simulink model "HEVminiproject"  (R2026a)
settings: configuration reference "VehicleVariable" (kept outside this file)
StartFcn:
  | %tic
StopFcn:
  | %toc
model workspace (MAT data in the model file):
  ExtDrvCmdsSwitch : Simulink.Parameter (value not decoded)
  ExtDrvRefSwitch : Simulink.Parameter (value not decoded)
  ExtEnvSwitch : Simulink.Parameter (value not decoded)
  ExtGndSwitch : Simulink.Parameter (value not decoded)
symbols that are objects in the model workspace (value not decoded): ExtDrvCmdsSwitch, ExtDrvRefSwitch, ExtEnvSwitch, ExtGndSwitch
undefined symbols (not defined in the file): AmbTemp, BaroPress, CtrlTcuInitGear, CurvGradRef, CurvRef, DCM, DriverAeroRes, DriverDrivelineRes, DriverInitialGear, DriverPreviewDist, DriverRollRes, DriverShiftTime, DriverTimeConst, DriverTractiveForce, EnvAbsPrs, EnvAirTemp, EnvGrvty, EnvNomFrictionScaling, EnvNominalGrade, EnvScnFrictionMap, EnvScnFrictionMapXBpts, EnvScnFrictionMapYBpts, EnvScnHeightMap, EnvScnHeightMapXBpts, EnvScnHeightMapYBpts, EnvWindVelX, EnvWindVelY, EnvWindVelZ, Gnd, Grade, HazzardCmd, HighBeamCmd, lambda_mux, LeftSignalCmd, LngRef, LowBeamCmd, LtrRef, PhiRef, PlntThrCabRelHInit, PlntThrRefrigPinit, PlntVehDstCGRearAxl, PlntVehInitYawAng, PlntVehMass, PlntVehTrckWdth, PlntVehYawMomentInertia, PlntWhlLdRadiusFrnt, PlntWhlLdRadiusRear, PsiRef, RightSignalCmd, Sim3dSensor, Wind, XRef, YRef, Z
libraries: simulink x28, autolibutils x5, autolibsharedcommon x5, vehdynlibviscommon x4, vehdynlibdriver x2, sim3dgroundtruthsensorlib x2, autolibshared x2, sl3dlib x1, sharedtransform x1, sim3dlib x1
(part 4 of 5)

== system HEVminiproject/Environment/Varying Friction/Varying Friction ==
  InertFrm : Inport
  Cg : Inport  Port=2
  Bus Creator2 : BusCreator  Inputs=4
  Bus Selector : BusSelector  OutputSignals=FrntAxl.Lft.Disp.X,FrntAxl.Rght.Disp.X,RearAxl.Lft.Disp.X,RearAxl.Rght.Disp.X
  Bus Selector1 : BusSelector  OutputSignals=FrntAxl.Lft.Disp.Y,FrntAxl.Rght.Disp.Y,RearAxl.Lft.Disp.Y,RearAxl.Rght.Disp.Y
  Demux1 : Demux
  Road Track Friction : Subsystem  mask(Road Track Friction){surface_popup=Split friction coefficient scaling factor, lambda_g=EnvNomFrictionScaling, lambda_r=.6, r_x0=175, r_y0=-100, r_xw=1000, r_yw=500, aMode=2}
      mask prompts: surface_popup "Type of surface:"; lambda_g "Scaling factor for the friction coefficient of ground, lambda_g :"; lambda_r "Scaling factor for the friction coefficient of rectangular surface, lambda_r :"; r_x0 "X coordinate of lower left corner of rectangular surface, r_x0 [m]:"; r_y0 "Y coordinate of lower left corner of rectangular surface, r_y0 [m]:"; r_xw "Rectangular surface width in X direction, r_xw [m]:"; r_yw "Rectangular surface width in Y direction, r_yw [m]:"
      mask init:
      | % Scaling factor for the friction coefficient around the rectangular region
      | mutable = [lambda_g, lambda_g, lambda_g, lambda_g;
      |            lambda_g, lambda_r, lambda_r, lambda_g; 
      |            lambda_g, lambda_r, lambda_r, lambda_g; 
      |            lambda_g, lambda_g, lambda_g, lambda_g ];
      |        
      | 
      | % The step is distance between breakpoint near the boundary of high and
      | % low friction coefficient
      | 
      | step = 0.01 ; 
      | 
      | % In the mask initialization, xbr and ybr breakpoints are with respect to
      | % Body fixed coordinate system. At time t=0, xbr and ybr breakpoints
      | % updates to Earth (Inertial) Fixed coordinate system. The breakpoints for
      | % the lookup table are added via inputs.
      | 
      | xbr = [(r_x0 - step) , (r_x0 + step), (r_x0 + r_xw - step) , (r_x0 + r_xw + step) ];
      | ybr = [(r_y0 - step) , (r_y0 + step), (r_y0 + r_yw - step) , (r_y0 + r_yw + step) ];
      | 
      | 
      | % To check if the created track is split mu or constant mu
      | 
      | surface_popup = get_param(gcb, 'surface_popup');
      | 
      | if strcmp(surface_popup, 'Split friction coefficient scaling factor')
      |     SplitLambdaTrck = 1;
      | elseif strcmp(surface_popup, 'Constant friction coefficient scaling factor')
      |     SplitLambdaTrck = 0;
      | end
      mask Help: eval('vdynblkshelp(''vdynblkstrack'')');
      mask TypeOptions surface_popup: Constant friction coefficient scaling factor | Split friction coefficient scaling factor
      mask Callback surface_popup:
      | surface_popup = get_param(gcb, 'surface_popup');
      | m = Simulink.Mask.get(gcb);
      | 
      | lambda_g = m.getParameter('lambda_g');
      | lambda_r = m.getParameter('lambda_r');
      | r_x0 = m.getParameter('r_x0');
      | r_y0 = m.getParameter('r_y0');
      | r_xw = m.getParameter('r_xw');
      | r_yw = m.getParameter('r_yw');
      | %track_view = m.getParameter('track_view');
      | 
      | 
      | if strcmp(surface_popup, 'Split friction coefficient scaling factor')
      |     lambda_g.Visible = 'on';
      |     lambda_r.Visible = 'on';
      |     r_x0.Visible = 'on';
      |     r_y0.Visible = 'on';
      |     r_xw.Visible = 'on';
      |     r_yw.Visible = 'on';
      |     %track_view.Visible = 'on';
      | 
      | elseif strcmp(surface_popup,'Constant friction coefficient scaling factor')
      |     lambda_g.Visible = 'on';
      |     lambda_r.Visible = 'off';
      |     r_x0.Visible = 'off';
      |     r_y0.Visible = 'off';
      |     r_xw.Visible = 'off';
      |     r_yw.Visible = 'off';
      |     %track_view.Visible = 'off';
      | end
      | [~]=autosharedicon('autolibutils',gcb,0);
      mask DialogControl DescGroupVar Prompt: Track description  (mask)
      mask DialogControl DescTextVar Prompt: Generates a default or user-specified track which creates a rectangular surface of specified friction coefficient. The location of rectangular surface is relative to the origin of Body Fixed Coordinate System.The input of the block is X and Y coordinates of the wheel from the vehicle feedback bus. The block output is friction coefficient for all the wheels.
  Wheel Coordinates : Subsystem
  mu : Outport
  wires:
  Bus Selector1/1 -> Wheel Coordinates/5(FrntAxlLftY)  "<Y>"
  Bus Selector/3 -> Wheel Coordinates/3(RearAxlLftX)  "<X>"
  Bus Selector/4 -> Wheel Coordinates/4(RearAxlRghtX)  "<X>"
  Wheel Coordinates/1(XWhl) -> Road Track Friction/1(XWhl)
  Bus Selector1/2 -> Wheel Coordinates/6(FrntAxlRghtY)  "<Y>"
  Bus Selector/2 -> Wheel Coordinates/2(FrntAxlRghtX)  "<X>"
  Bus Selector/1 -> Wheel Coordinates/1(FrntAxlLftX)  "<X>"
  Bus Selector1/3 -> Wheel Coordinates/7(RearAxlLftY)  "<Y>"
  Bus Selector1/4 -> Wheel Coordinates/8(RearAxlRghtY)  "<Y>"
  Cg/1 -> Road Track Friction/3(Cg)
  Wheel Coordinates/2(YWhl) -> Road Track Friction/2(YWhl)
  InertFrm/1 -> Bus Selector1/1, Bus Selector/1
  Road Track Friction/1(FricCoeffLambda) -> Demux1/1
  Demux1/1 -> Bus Creator2/1  "mu_FL"
  Demux1/4 -> Bus Creator2/4  "mu_RR"
  Demux1/2 -> Bus Creator2/2  "mu_FR"
  Demux1/3 -> Bus Creator2/3  "mu_RL"
  Bus Creator2/1 -> mu/1  "mu"

== system HEVminiproject/Scenarios/Coordinate Systems/ISO 8855 (Z-up) ==
  ExtDrvRefIn : Inport
  ExtDrvCmdIn : Inport  Port=2
  Bus Assignment : BusAssignment  AssignedSignals=LtrRef,YRef,PhiRef,CurvRef,CurvGradRef
  Bus Assignment1 : BusAssignment  AssignedSignals=SteerCmd.SteerCmd
  Bus Selector : BusSelector  OutputSignals=LtrRef,YRef,PhiRef,CurvRef,CurvGradRef
  Bus Selector1 : BusSelector  OutputSignals=SteerCmd.SteerCmd
  Unary Minus{,1..5} (6 alike) : UnaryMinus
  ExtDrvRef : Outport
  ExtDrvCmd : Outport  Port=2
  wires:
  ExtDrvRefIn/1 -> Bus Assignment/1, Bus Selector/1
  ExtDrvCmdIn/1 -> Bus Assignment1/1, Bus Selector1/1
  Unary Minus/1 -> Bus Assignment/2
  Bus Assignment1/1 -> ExtDrvCmd/1
  Bus Assignment/1 -> ExtDrvRef/1
  Bus Selector/1 -> Unary Minus/1  "<LtrRef>"
  Unary Minus2/1 -> Bus Assignment/3
  Unary Minus3/1 -> Bus Assignment/4
  Unary Minus4/1 -> Bus Assignment/5
  Unary Minus5/1 -> Bus Assignment/6
  Bus Selector/2 -> Unary Minus2/1  "<YRef>"
  Bus Selector/3 -> Unary Minus3/1  "<PhiRef>"
  Bus Selector/4 -> Unary Minus4/1  "<CurvRef>"
  Bus Selector/5 -> Unary Minus5/1  "<CurvGradRef>"
  Unary Minus1/1 -> Bus Assignment1/2
  Bus Selector1/1 -> Unary Minus1/1  "<SteerCmd>"

== system HEVminiproject/Scenarios/Coordinate Systems/SAE J670 (Z-down) ==
  ExtDrvRefIn : Inport
  ExtDrvCmdIn : Inport  Port=2
  ExtDrvRef : Outport
  ExtDrvCmd : Outport  Port=2
  wires:
  ExtDrvCmdIn/1 -> ExtDrvCmd/1
  ExtDrvRefIn/1 -> ExtDrvRef/1

== system HEVminiproject/Scenarios/Reference Generator/Drive Cycle ==
  "VehFdbk " : Inport
  Bus Assignment : BusAssignment  AssignedSignals=LngRef,XRef
  Bus Creator : BusCreator  Inputs=3
  Bus Selector : BusSelector  OutputSignals=Body.InertFrm.Cg.Disp.X
  Constant13 : Constant  Value=0
  Constant14 : Constant  Value=0
  Constant15 : Constant  Value=0
  Drive Cycle Source : autolibshared/Drive Cycle Source  cycleVar=FTP75  fileVar=L:\Bauto\matlab\test\toolbox\shared\autoblks\scenario\adac.txt  tfinal="2474  seconds"  cycleRepeat=off  outAccPort=off  outGearPort=off  gearList=No gear data  t_wot1=t_start  xdot_woto=0  xdot_wot1=xdot_r  t_wot2=t_wot2  xdot_wot2=0  t_wotend=ScnSimTime  srcUnit=m/s  outUnit=mph  srcAccUnit=m/s/s  outAccUnit=m/s^2  dt=0  aMode=6  faultOption=off  velBnd=2  velBndUnit=mph  inUnit=m/s  timeBnd=1  failOption=off  stopSim=off  maxFaultCnt=10  maxFaultTime=2  maxTotFaultTime=15  traceOption=off  dtTrace=1  traceWindow=10  lastDCname=FTP75  lastOutUnit=mph  lastDT=0  lastTB=1  lastSB=2  forceCalcBound=off
  DrvCmdSrc : autolibsharedcommon/DrvCmd  SystemSampleTime=-1  VariantActivationTime=update diagram  EmptyChoice=off  PassThrough=off  PassThroughVariantControl=(default)  EmptyChoiceVariantControl=(default)  AllowFlexibleInterface=on  Latency=0  AutoFrameSizeCalculation=off
  DrvRefSrc : autolibsharedcommon/DrvRef  SystemSampleTime=-1  VariantActivationTime=update diagram  EmptyChoice=off  PassThrough=off  PassThroughVariantControl=(default)  EmptyChoiceVariantControl=(default)  AllowFlexibleInterface=on  Latency=0  AutoFrameSizeCalculation=off
  Unit Conversion : UnitConversion
  " Vis" : Outport  VectorParamsAs1DForOutWhenUnconnected=off
  DrvRef : Outport  Port=2  VectorParamsAs1DForOutWhenUnconnected=off
  DrvCmd : Outport  Port=3  VectorParamsAs1DForOutWhenUnconnected=off
  " Fdbk" : Outport  Port=4  VectorParamsAs1DForOutWhenUnconnected=off
  wires:
  Constant13/1 -> Bus Creator/1  "XRef"
  Constant14/1 -> Bus Creator/2  "YRef"
  Constant15/1 -> Bus Creator/3  "ZRef"
  Bus Creator/1 -> " Vis"/1
  Drive Cycle Source/1 -> Unit Conversion/1
  Bus Selector/1 -> Bus Assignment/3  "<X>"
  "VehFdbk "/1 -> Bus Selector/1, " Fdbk"/1
  DrvRefSrc/1 -> Bus Assignment/1
  Bus Assignment/1 -> DrvRef/1
  DrvCmdSrc/1 -> DrvCmd/1
  Unit Conversion/1 -> Bus Assignment/2

== system HEVminiproject/Scenarios/Reference Generator/WOT ==
  "VehFdbk " : Inport
  Bus Assignment : BusAssignment  AssignedSignals=LngRef,XRef,YRef,PsiRef
  Bus Creator : BusCreator  Inputs=3
  Bus Selector : BusSelector  OutputSignals=Body.InertFrm.Cg.Disp.X,Body.InertFrm.Cg.Disp.Y,Body.InertFrm.Cg.Ang.psi
  Constant13 : Constant  Value=0
  Constant14 : Constant  Value=0
  Constant15 : Constant  Value=0
  Drive Cycle Source : autolibshared/Drive Cycle Source  cycleVar=Wide Open Throttle (WOT)  fileVar=L:\Bauto\matlab\test\toolbox\shared\autoblks\scenario\adac.txt  tfinal="40  seconds"  cycleRepeat=off  outAccPort=off  outGearPort=off  gearList=No gear data  t_wot1=ScnStartTime  xdot_woto=0  xdot_wot1=ScnLongVelRef  t_wot2=ScnTimeToStrtDecel  xdot_wot2=0  t_wotend=40  srcUnit=mph  outUnit=mph  srcAccUnit=m/s/s  outAccUnit=m/s^2  dt=0  aMode=6  faultOption=off  velBnd=2  velBndUnit=mph  inUnit=m/s  timeBnd=1  failOption=off  stopSim=off  maxFaultCnt=10  maxFaultTime=2  maxTotFaultTime=15  traceOption=off  dtTrace=1  traceWindow=10  lastDCname=Custom Data Set  lastOutUnit=mph  lastDT=0  lastTB=1  lastSB=2  forceCalcBound=off
  DrvCmdSrc : autolibsharedcommon/DrvCmd  SystemSampleTime=-1  VariantActivationTime=update diagram  EmptyChoice=off  PassThrough=off  PassThroughVariantControl=(default)  EmptyChoiceVariantControl=(default)  AllowFlexibleInterface=on  Latency=0  AutoFrameSizeCalculation=off
  DrvRefSrc : autolibsharedcommon/DrvRef  SystemSampleTime=-1  VariantActivationTime=update diagram  EmptyChoice=off  PassThrough=off  PassThroughVariantControl=(default)  EmptyChoiceVariantControl=(default)  AllowFlexibleInterface=on  Latency=0  AutoFrameSizeCalculation=off
  Unit Conversion : UnitConversion
  " Vis" : Outport  VectorParamsAs1DForOutWhenUnconnected=off
  " Fdbk" : Outport  Port=2  VectorParamsAs1DForOutWhenUnconnected=off
  DrvRef : Outport  Port=3  VectorParamsAs1DForOutWhenUnconnected=off
  DrvCmd : Outport  Port=4  VectorParamsAs1DForOutWhenUnconnected=off
  wires:
  Drive Cycle Source/1 -> Unit Conversion/1
  Bus Creator/1 -> " Vis"/1
  Constant15/1 -> Bus Creator/3  "ZRef"
  Constant14/1 -> Bus Creator/2  "YRef"
  Constant13/1 -> Bus Creator/1  "XRef"
  Bus Selector/2 -> Bus Assignment/4  "<Y>"
  DrvRefSrc/1 -> Bus Assignment/1
  DrvCmdSrc/1 -> DrvCmd/1
  Bus Selector/1 -> Bus Assignment/3  "<X>"
  Bus Assignment/1 -> DrvRef/1
  Bus Selector/3 -> Bus Assignment/5  "<psi>"
  "VehFdbk "/1 -> Bus Selector/1, " Fdbk"/1
  Unit Conversion/1 -> Bus Assignment/2

== system HEVminiproject/Visualization/3D Engine/3D Engine Disabled ==
  VehFdbk : Inport
  Terminator : Terminator
  wires:
  VehFdbk/1 -> Terminator/1

== system HEVminiproject/Visualization/Coordinate Systems/ISO 8855 (Z-up) ==
  VehFdbkIn : Inport
  Bus Assignment : BusAssignment  AssignedSignals=Body.InertFrm.Cg.Disp.Y,Body.InertFrm.Cg.Disp.Z,Body.InertFrm.Cg.Vel.Ydot,Body.InertFrm.Cg.Vel.Zdot,Body.InertFrm.Geom.Disp.Y,Body.InertFrm.Geom.Disp.Z,Body.InertFrm.Cg.Ang.theta,Body.InertFrm.Cg.Ang.psi,Body.BdyFrm.Cg.Vel.ydot,Body.BdyFrm.Cg.Vel.zdot,Body.BdyFrm.Cg.AngVel.q,Body.BdyFrm.Cg.AngVel.r,Body.BdyFrm.Cg.Acc.ay,Body.BdyFrm.Cg.Acc.az,Body.BdyFrm.Cg.Acc.yddot,Body.BdyFrm.Cg.Acc.zddot
  Bus Selector : BusSelector  OutputSignals=Body.InertFrm.Cg.Disp.Y,Body.InertFrm.Cg.Disp.Z,Body.InertFrm.Cg.Vel.Ydot,Body.InertFrm.Cg.Vel.Zdot,Body.InertFrm.Geom.Disp.Y,Body.InertFrm.Geom.Disp.Z,Body.InertFrm.Cg.Ang.theta,Body.InertFrm.Cg.Ang.psi,Body.BdyFrm.Cg.Vel.ydot,Body.BdyFrm.Cg.Vel.zdot,Body.BdyFrm.Cg.AngVel.q,Body.BdyFrm.Cg.AngVel.r,Body.BdyFrm.Cg.Acc.ay,Body.BdyFrm.Cg.Acc.az,Body.BdyFrm.Cg.Acc.yddot,Body.BdyFrm.Cg.Acc.zddot
  Unary Minus{,1..15} (16 alike) : UnaryMinus
  VehFdbk : Outport
  wires:
  VehFdbkIn/1 -> Bus Assignment/1, Bus Selector/1
  Bus Assignment/1 -> VehFdbk/1
  Bus Selector/1 -> Unary Minus/1  "<Y>"
  Bus Selector/2 -> Unary Minus2/1  "<Z>"
  Bus Selector/11 -> Unary Minus10/1  "<q>"
  Bus Selector/12 -> Unary Minus11/1  "<r>"
  Bus Selector/13 -> Unary Minus12/1  "<ay>"
  Bus Selector/14 -> Unary Minus13/1  "<az>"
  Bus Selector/15 -> Unary Minus14/1  "<yddot>"
  Bus Selector/16 -> Unary Minus15/1  "<zddot>"
  Bus Selector/3 -> Unary Minus3/1  "<Ydot>"
  Bus Selector/4 -> Unary Minus4/1  "<Zdot>"
  Bus Selector/5 -> Unary Minus5/1  "<Y>"
  Bus Selector/6 -> Unary Minus1/1  "<Z>"
  Bus Selector/7 -> Unary Minus6/1  "<theta>"
  Bus Selector/8 -> Unary Minus7/1  "<psi>"
  Bus Selector/9 -> Unary Minus8/1  "<ydot>"
  Bus Selector/10 -> Unary Minus9/1  "<zdot>"
  Unary Minus/1 -> Bus Assignment/2
  Unary Minus2/1 -> Bus Assignment/3
  Unary Minus3/1 -> Bus Assignment/4
  Unary Minus4/1 -> Bus Assignment/5
  Unary Minus8/1 -> Bus Assignment/10
  Unary Minus9/1 -> Bus Assignment/11
  Unary Minus10/1 -> Bus Assignment/12
  Unary Minus11/1 -> Bus Assignment/13
  Unary Minus12/1 -> Bus Assignment/14
  Unary Minus13/1 -> Bus Assignment/15
  Unary Minus14/1 -> Bus Assignment/16
  Unary Minus15/1 -> Bus Assignment/17
  Unary Minus5/1 -> Bus Assignment/6
  Unary Minus1/1 -> Bus Assignment/7
  Unary Minus6/1 -> Bus Assignment/8
  Unary Minus7/1 -> Bus Assignment/9

== system HEVminiproject/Visualization/Coordinate Systems/SAE J670 (Z-down) ==
  VehFdbkIn : Inport
  VehFdbk : Outport
  wires:
  VehFdbkIn/1 -> VehFdbk/1

== system HEVminiproject/Visualization/ISO 15037-1:2006/Disabled ==
  VehFdbk : Inport
  Terminator1 : Terminator
  wires:
  VehFdbk/1 -> Terminator1/1

== system HEVminiproject/Visualization/ISO 15037-1:2006/Enabled ==
  VehFdbk : Inport
  Bus Selector : BusSelector  OutputSignals=Driver.SteerFdbk,Body.BdyFrm.Cg.Vel.xdot,Body.BdyFrm.Cg.Vel.ydot,Body.BdyFrm.Cg.Acc.ax,Body.BdyFrm.Cg.Acc.ay,Body.BdyFrm.Cg.AngVel.r,Body.BdyFrm.Cg.AngVel.q,Body.BdyFrm.Cg.AngVel.p,Body.InertFrm.Cg.Ang.phi,Body.InertFrm.Cg.Ang.theta
  Signal Specification : SignalSpecification  Unit=deg
  Signal Specification10 : SignalSpecification  Unit=deg
  Signal Specification11 : SignalSpecification  Unit=deg
  Signal Specification2 : SignalSpecification  Unit=km/h
  Signal Specification3 : SignalSpecification  Unit=m/s
  Signal Specification5 : SignalSpecification  Unit=m/s^2
  Signal Specification6 : SignalSpecification  Unit=m/s^2
  Signal Specification7 : SignalSpecification  Unit=deg/s
  Signal Specification8 : SignalSpecification  Unit=deg/s
  Signal Specification9 : SignalSpecification  Unit=deg/s
  Terminator{,2..3,5..11} (10 alike) : Terminator
  Unit Conversion{2..4,6..12} (10 alike) : UnitConversion
  wires:
  Bus Selector/10 -> Unit Conversion12/1  "<theta>"
  Signal Specification11/1 -> Terminator11/1  "Pitch angle"
  Unit Conversion12/1 -> Signal Specification11/1
  Bus Selector/9 -> Unit Conversion11/1  "<phi>"
  Unit Conversion11/1 -> Signal Specification10/1
  Signal Specification10/1 -> Terminator10/1  "Roll angle"
  Bus Selector/8 -> Unit Conversion10/1  "<p>"
  Signal Specification9/1 -> Terminator9/1  "Roll velocity"
  Unit Conversion10/1 -> Signal Specification9/1
  Bus Selector/7 -> Unit Conversion9/1  "<q>"
  Unit Conversion9/1 -> Signal Specification8/1
  Signal Specification8/1 -> Terminator8/1  "Pitch velocity"
  Bus Selector/6 -> Unit Conversion8/1  "<r>"
  Signal Specification7/1 -> Terminator7/1  "Yaw velocity"
  Unit Conversion8/1 -> Signal Specification7/1
  Bus Selector/5 -> Unit Conversion7/1  "<ay>"
  Unit Conversion7/1 -> Signal Specification6/1
  Signal Specification6/1 -> Terminator6/1  "Lateral acceleration"
  Bus Selector/4 -> Unit Conversion6/1  "<ax>"
  Signal Specification5/1 -> Terminator5/1  "Longitudinal acceleration"
  Unit Conversion6/1 -> Signal Specification5/1
  Bus Selector/3 -> Unit Conversion4/1  "<ydot>"
  Signal Specification3/1 -> Terminator3/1  "Lateral velocity"
  Unit Conversion4/1 -> Signal Specification3/1
  Bus Selector/2 -> Unit Conversion3/1  "<xdot>"
  Unit Conversion3/1 -> Signal Specification2/1
  Signal Specification2/1 -> Terminator2/1  "Longitudinal velocity"
  Signal Specification/1 -> Terminator/1  "Steering-wheel angle"
  Unit Conversion2/1 -> Signal Specification/1
  VehFdbk/1 -> Bus Selector/1
  Bus Selector/1 -> Unit Conversion2/1  "<SteerFdbk>"

== system HEVminiproject/Visualization/Scope Type/DLC ==
  VehFdbk : Inport
  Vis : Inport  Port=2
  Bus Creator : BusCreator  Inputs=3
  Bus Selector3 : BusSelector  OutputSignals=Body.InertFrm.Cg.Disp.X,Body.InertFrm.Cg.Disp.Z
  Bus Selector4 : BusSelector  OutputSignals=LeftBnd,RightBnd,LtrlRef
  Lane Change : Scope
      settings: Title=Double Lane Change: Lateral Displacement  ActiveDisplayYMinimum=-3.28469  ActiveDisplayYMaximum=6.06905  YLabel=Lateral Displacement [m] (positive = right direction)  DataLoggingSaveFormat=Array
  Mux1 : Mux  Inputs=3
  Rate Transition : RateTransition  OutPortSampleTime=.1
  Rate Transition1 : RateTransition  OutPortSampleTime=.1
  Rate Transition3 : RateTransition  OutPortSampleTime=.1
  Signal Copy : SignalConversion  OverrideOpt=off
  Signal Copy1 : SignalConversion  OverrideOpt=off
  Signal Copy2 : SignalConversion  OverrideOpt=off
  Ref : Outport  VectorParamsAs1DForOutWhenUnconnected=off
  wires:
  VehFdbk/1 -> Bus Selector3/1
  Vis/1 -> Bus Selector4/1
  Bus Creator/1 -> Ref/1
  Bus Selector3/2 -> Signal Copy2/1  "<Z>"
  Signal Copy/1 -> Bus Creator/2  "YRef"
  Signal Copy1/1 -> Bus Creator/1  "XRef"
  Signal Copy2/1 -> Bus Creator/3  "ZRef"
  Rate Transition3/1 -> Mux1/2  "Right Boundary"
  Bus Selector4/3 -> Signal Copy/1, Rate Transition1/1  "<LtrlRef>"
  Mux1/1 -> Lane Change/1
  Bus Selector4/1 -> Rate Transition/1  "<LeftBnd>"
  Rate Transition/1 -> Mux1/1  "Left Boundary"
  Bus Selector4/2 -> Rate Transition3/1  "<RightBnd>"
  Bus Selector3/1 -> Signal Copy1/1  "<X>"
  Rate Transition1/1 -> Mux1/3  "Reference"

== system HEVminiproject/Visualization/Scope Type/None ==
  VehFdbk : Inport
  Vis : Inport  Port=2
  Bus Selector2 : BusSelector  OutputSignals=Driver.SteerFdbk
  Bus Selector9 : BusSelector  OutputSignals=Body.BdyFrm.Cg.AngVel.r
  Signal Specification1 : SignalSpecification  Unit=rad/s
  Signal Specification3 : SignalSpecification  Unit=deg/s
  Unit Conversion4 : UnitConversion
  Yaw Rate and Steer : Scope  NumInputPorts=2
      settings: ActiveDisplayYMinimum=-112.49987  ActiveDisplayYMaximum=112.49996
  Ref : Outport  VectorParamsAs1DForOutWhenUnconnected=off
  wires:
  Bus Selector9/1 -> Signal Specification1/1  "<r>"
  Signal Specification3/1 -> Yaw Rate and Steer/1
  Unit Conversion4/1 -> Signal Specification3/1
  VehFdbk/1 -> Bus Selector2/1, Bus Selector9/1  "VehFdbk"
  Bus Selector2/1 -> Yaw Rate and Steer/2  "<SteerFdbk>"
  Vis/1 -> Ref/1
  Signal Specification1/1 -> Unit Conversion4/1

== system HEVminiproject/Visualization/Scope Type/XYZ ==
  VehFdbk : Inport
  Vis : Inport  Port=2
  Terminator : Terminator
  Ref : Outport  VectorParamsAs1DForOutWhenUnconnected=off
  wires:
  Vis/1 -> Ref/1
  VehFdbk/1 -> Terminator/1

== system HEVminiproject/Visualization/Vehicle XY Plotter/Disabled ==

== system HEVminiproject/Visualization/Vehicle XY Plotter/XY View ==
  Bus Element In2 : Inport  PortName=VehFdbk
  Bus Selector1 : BusSelector  OutputSignals=Body.InertFrm.Cg.Ang.phi,Body.InertFrm.Cg.Ang.theta,Body.InertFrm.Cg.Ang.psi  OutputAsBus=on
  Bus Selector10 : BusSelector  OutputSignals=FrntWheels.Wheels.Fx,RearWheels.Wheels.Fx,FrntWheels.Wheels.Fy,RearWheels.Wheels.Fy
  Bus Selector5 : BusSelector  OutputSignals=Steering.Front.WhlAng.FL,Steering.Front.WhlAng.FR,Steering.Rear.WhlAng.RL,Steering.Rear.WhlAng.RR  OutputAsBus=on
  Bus Selector6 : BusSelector  OutputSignals=Body.InertFrm.Geom.Disp.X,Body.InertFrm.Geom.Disp.Y,Body.InertFrm.Geom.Disp.Z  OutputAsBus=on
  Bus Selector7 : BusSelector  OutputSignals=Body.InertFrm.Geom.Vel.Xdot,Body.InertFrm.Geom.Vel.Ydot,Body.InertFrm.Geom.Vel.Zdot  OutputAsBus=on
  Bus Selector9 : BusSelector  OutputSignals=Trans.Info.Eng.EngSpd,EM.EMSpd,Trans.Info.Trans.TransGear
  Bus to Vector{,1..2,4..6} (6 alike) : BusToVector
  Driveline Speed : Subsystem
  Vector Concatenate : Concatenate
  Vector Concatenate1 : Concatenate
  Vector Concatenate2 : Concatenate
  Vehicle XY Plotter : vehdynlibviscommon/Vehicle XY Plot Configuration  extRef=off  extStats=on  extTireF=on  a=PlntVehDstCGFrntAxl  b=PlntVehDstCGRearAxl  w=PlntVehTrckWdth(1)  figBorder=10  bufferSize=1024  velNorm=5  tireFNorm=1000  tireFMin=20  pltDT=.1
  wires:
  Bus Selector7/1 -> Bus to Vector1/1
  Bus Selector5/1 -> Bus to Vector4/1
  Bus to Vector1/1 -> Vehicle XY Plotter/3
  Bus Selector1/1 -> Bus to Vector2/1
  Vector Concatenate2/1 -> Vehicle XY Plotter/5
  Bus to Vector/1 -> Vehicle XY Plotter/1
  Bus Selector6/1 -> Bus to Vector/1
  Bus to Vector2/1 -> Vehicle XY Plotter/2
  Bus Element In2/1 -> Bus Selector5/1, Bus Selector10/1, Bus Selector9/1, Bus Selector7/1, Bus Selector1/1, Bus Selector6/1  "VehFdbk"
  Bus to Vector4/1 -> Vehicle XY Plotter/4
  Bus Selector10/2 -> Bus to Vector6/1  "<Fx>"
  Vector Concatenate1/1 -> Vehicle XY Plotter/7
  Vector Concatenate/1 -> Vehicle XY Plotter/6
  Bus Selector10/1 -> Bus to Vector5/1  "<Fx>"
  Bus Selector10/3 -> Vector Concatenate1/1  "<Fy>"
  Bus Selector10/4 -> Vector Concatenate1/2  "<Fy>"
  Bus to Vector5/1 -> Vector Concatenate/1
  Bus to Vector6/1 -> Vector Concatenate/2
  Bus Selector9/3 -> Vector Concatenate2/2  "<TransGear>"
  Bus Selector9/2 -> Driveline Speed/2(<EMSpd>)  "<EMSpd>"
  Driveline Speed/1(MaxSpd) -> Vector Concatenate2/1
  Bus Selector9/1 -> Driveline Speed/1(<EngSpd>)  "<EngSpd>"

== system HEVminiproject/Visualization/Vehicle XY Plotter/XY View Ref ==
  Bus Element In2 : Inport  PortName=VehFdbk
  Bus Element In1 : Inport  Port=2  PortName=Ref  Element=YRef
  Bus Element In3 : Inport  Port=2  PortName=Ref  Element=XRef
  Bus Selector1 : BusSelector  OutputSignals=Body.InertFrm.Cg.Ang.phi,Body.InertFrm.Cg.Ang.theta,Body.InertFrm.Cg.Ang.psi  OutputAsBus=on
  Bus Selector10 : BusSelector  OutputSignals=FrntWheels.Wheels.Fx,RearWheels.Wheels.Fx,FrntWheels.Wheels.Fy,RearWheels.Wheels.Fy
  Bus Selector5 : BusSelector  OutputSignals=Steering.Front.WhlAng.FL,Steering.Front.WhlAng.FR,Steering.Rear.WhlAng.RL,Steering.Rear.WhlAng.RR  OutputAsBus=on
  Bus Selector6 : BusSelector  OutputSignals=Body.InertFrm.Geom.Disp.X,Body.InertFrm.Geom.Disp.Y,Body.InertFrm.Geom.Disp.Z  OutputAsBus=on
  Bus Selector7 : BusSelector  OutputSignals=Body.InertFrm.Geom.Vel.Xdot,Body.InertFrm.Geom.Vel.Ydot,Body.InertFrm.Geom.Vel.Zdot  OutputAsBus=on
  Bus Selector9 : BusSelector  OutputSignals=Trans.Info.Eng.EngSpd,EM.EMSpd,Trans.Info.Trans.TransGear
  Bus to Vector{,1..2,4..5} (5 alike) : BusToVector
  Driveline Speed : Subsystem
  Ground1 : Ground
  Mux : Mux  Inputs=3
  Vector Concatenate : Concatenate
  Vector Concatenate1 : Concatenate
  Vector Concatenate2 : Concatenate
  Vehicle XY Plotter : vehdynlibviscommon/Vehicle XY Plot Configuration  extRef=on  extStats=on  extTireF=on  a=PlntVehDstCGFrntAxl  b=PlntVehDstCGRearAxl  w=PlntVehTrckWdth(1)  figBorder=10  bufferSize=1024  velNorm=5  tireFNorm=1000  tireFMin=20  pltDT=.1
  wires:
  Bus Selector7/1 -> Bus to Vector1/1
  Bus Selector5/1 -> Vehicle XY Plotter/4
  Ground1/1 -> Mux/3
  Bus to Vector1/1 -> Vehicle XY Plotter/3
  Bus Selector1/1 -> Bus to Vector2/1
  Bus Element In1/1 -> Mux/2
  Bus Element In3/1 -> Mux/1
  Mux/1 -> Vehicle XY Plotter/5
  Bus to Vector/1 -> Vehicle XY Plotter/1
  Bus Selector6/1 -> Bus to Vector/1
  Bus to Vector2/1 -> Vehicle XY Plotter/2
  Bus Selector10/1 -> Bus to Vector4/1  "<Fx>"
  Bus Selector10/2 -> Bus to Vector5/1  "<Fx>"
  Bus Selector10/4 -> Vector Concatenate1/2  "<Fy>"
  Vector Concatenate/1 -> Vehicle XY Plotter/7
  Bus Selector10/3 -> Vector Concatenate1/1  "<Fy>"
  Vector Concatenate1/1 -> Vehicle XY Plotter/8
  Bus to Vector4/1 -> Vector Concatenate/1
  Bus to Vector5/1 -> Vector Concatenate/2
  Driveline Speed/1(MaxSpd) -> Vector Concatenate2/1
  Bus Selector9/2 -> Driveline Speed/2(<EMSpd>)  "<EMSpd>"
  Bus Selector9/1 -> Driveline Speed/1(<EngSpd>)  "<EngSpd>"
  Bus Element In2/1 -> Bus Selector5/1, Bus Selector7/1, Bus Selector1/1, Bus Selector6/1, Bus Selector9/1, Bus Selector10/1  "VehFdbk"
  Bus Selector9/3 -> Vector Concatenate2/2  "<TransGear>"
  Vector Concatenate2/1 -> Vehicle XY Plotter/6

== system HEVminiproject/Visualization/Vehicle XY Plotter/XY View Ref with One-Axle Trailer ==
  Bus Element In2 : Inport  PortName=VehFdbk
  Bus Element In1 : Inport  Port=2  PortName=Ref  Element=YRef
  Bus Element In3 : Inport  Port=2  PortName=Ref  Element=XRef
  Bus Selector1 : BusSelector  OutputSignals=Body.InertFrm.Cg.Ang.phi,Body.InertFrm.Cg.Ang.theta,Body.InertFrm.Cg.Ang.psi  OutputAsBus=on
  Bus Selector10 : BusSelector  OutputSignals=FrntWheels.Wheels.Fx,RearWheels.Wheels.Fx,FrntWheels.Wheels.Fy,RearWheels.Wheels.Fy,TrlrWheels.Wheels.TireFrame.Fx,TrlrWheels.Wheels.TireFrame.Fy
  Bus Selector16 : BusSelector  OutputSignals=TrlrWheels.Wheels.Steering.WheelAngles  OutputAsBus=on
  Bus Selector2 : BusSelector  OutputSignals=TrlrBody.InertFrm.Geom.Disp.X,TrlrBody.InertFrm.Geom.Disp.Y,TrlrBody.InertFrm.Geom.Disp.Z  OutputAsBus=on
  Bus Selector3 : BusSelector  OutputSignals=TrlrBody.InertFrm.Cg.Ang.phi,TrlrBody.InertFrm.Cg.Ang.theta,TrlrBody.InertFrm.Cg.Ang.psi  OutputAsBus=on
  Bus Selector4 : BusSelector  OutputSignals=TrlrBody.InertFrm.Geom.Vel.Xdot,TrlrBody.InertFrm.Geom.Vel.Ydot,TrlrBody.InertFrm.Geom.Vel.Zdot  OutputAsBus=on
  Bus Selector5 : BusSelector  OutputSignals=Steering.Front.WhlAng.FL,Steering.Front.WhlAng.FR,Steering.Rear.WhlAng.RL,Steering.Rear.WhlAng.RR  OutputAsBus=on
  Bus Selector6 : BusSelector  OutputSignals=Body.InertFrm.Geom.Disp.X,Body.InertFrm.Geom.Disp.Y,Body.InertFrm.Geom.Disp.Z  OutputAsBus=on
  Bus Selector7 : BusSelector  OutputSignals=Body.InertFrm.Geom.Vel.Xdot,Body.InertFrm.Geom.Vel.Ydot,Body.InertFrm.Geom.Vel.Zdot  OutputAsBus=on
  Bus Selector8 : BusSelector  OutputSignals=Trans.Info.Eng.EngSpd,EM.EMSpd,Trans.Info.Trans.TransGear
  Bus to Vector{,1..2,4..9} (9 alike) : BusToVector
  Driveline Speed : Subsystem
  Ground1 : Ground
  Mux : Mux  Inputs=3
  Vector Concatenate : Concatenate
  Vector Concatenate1 : Concatenate
  Vector Concatenate2 : Concatenate
  Vehicle XY Plot Configuration with One-Axle Trailer : vehdynlibviscommon/Vehicle XY Plot Configuration with One-Axle Trailer  extRef=on  extStats=on  extTireF=on  a=PlntVehDstCGFrntAxl  b=PlntVehDstCGRearAxl  w=PlntVehTrckWdth(1)  figBorder=10  bufferSize=1024  velNorm=5  tireFNorm=1000  pltDT=.1
  wires:
  Bus Selector10/4 -> Vector Concatenate1/2  "<Fy>"
  Bus Selector10/1 -> Bus to Vector8/1  "<Fx>"
  Bus Selector10/2 -> Bus to Vector9/1  "<Fx>"
  Bus Selector2/1 -> Bus to Vector4/1
  Vector Concatenate2/1 -> Vehicle XY Plot Configuration with One-Axle Trailer/6
  Bus Selector16/1 -> Bus to Vector7/1
  Bus to Vector/1 -> Vehicle XY Plot Configuration with One-Axle Trailer/1
  Bus to Vector6/1 -> Vehicle XY Plot Configuration with One-Axle Trailer/12
  Ground1/1 -> Mux/3
  Bus Selector7/1 -> Bus to Vector1/1
  Bus Selector4/1 -> Bus to Vector5/1
  Bus to Vector7/1 -> Vehicle XY Plot Configuration with One-Axle Trailer/14
  Bus to Vector4/1 -> Vehicle XY Plot Configuration with One-Axle Trailer/11
  Vector Concatenate1/1 -> Vehicle XY Plot Configuration with One-Axle Trailer/8
  Bus to Vector5/1 -> Vehicle XY Plot Configuration with One-Axle Trailer/13
  Bus Selector10/6 -> Vehicle XY Plot Configuration with One-Axle Trailer/10  "<Fy>"
  Bus Selector3/1 -> Bus to Vector6/1
  Bus Selector6/1 -> Bus to Vector/1
  Mux/1 -> Vehicle XY Plot Configuration with One-Axle Trailer/5
  Bus Selector1/1 -> Bus to Vector2/1
  Bus Element In1/1 -> Mux/2
  Bus Selector10/5 -> Vehicle XY Plot Configuration with One-Axle Trailer/9  "<Fx>"
  Bus Element In3/1 -> Mux/1
  Bus Selector10/3 -> Vector Concatenate1/1  "<Fy>"
  Vector Concatenate/1 -> Vehicle XY Plot Configuration with One-Axle Trailer/7
  Bus Selector5/1 -> Vehicle XY Plot Configuration with One-Axle Trailer/4
  Bus to Vector1/1 -> Vehicle XY Plot Configuration with One-Axle Trailer/3
  Bus to Vector2/1 -> Vehicle XY Plot Configuration with One-Axle Trailer/2
  Bus to Vector8/1 -> Vector Concatenate/1
  Bus to Vector9/1 -> Vector Concatenate/2
  Driveline Speed/1(MaxSpd) -> Vector Concatenate2/1
  Bus Selector8/2 -> Driveline Speed/2(<EMSpd>)  "<EMSpd>"
  Bus Selector8/1 -> Driveline Speed/1(<EngSpd>)  "<EngSpd>"
  Bus Element In2/1 -> Bus Selector10/1, Bus Selector4/1, Bus Selector16/1, Bus Selector3/1, Bus Selector2/1, Bus Selector8/1, Bus Selector5/1, Bus Selector7/1, Bus Selector1/1, Bus Selector6/1  "VehFdbk"
  Bus Selector8/3 -> Vector Concatenate2/2  "<TransGear>"

== system HEVminiproject/Driver Commands/Driver Commands/Dashboard Widgets/Widget Sinks ==
  VehFdbk : Inport
  Bus Selector : BusSelector  OutputSignals=Driver.LightsFdbk.HighBeamFdbk,Driver.LightsFdbk.LowBeamFdbk,Driver.LightsFdbk.LeftSignalFdbk,Driver.LightsFdbk.RightSignalFdbk,Driver.LightsFdbk.HazzardFdbk
  Terminator{,1..4} (5 alike) : Terminator
  wires:
  Bus Selector/5 -> Terminator4/1  "<HazzardFdbk>"
  Bus Selector/3 -> Terminator2/1  "<LeftSignalFdbk>"
  Bus Selector/4 -> Terminator3/1  "<RightSignalFdbk>"
  Bus Selector/2 -> Terminator1/1  "<LowBeamFdbk>"
  Bus Selector/1 -> Terminator/1  "<HighBeamFdbk>"
  VehFdbk/1 -> Bus Selector/1

== system HEVminiproject/Driver Commands/Driver Commands/Dashboard Widgets/Widget Sources ==
  Accelerator : Constant  Value=0  SampleTime=-1
  Brake : Constant  Value=0  SampleTime=-1
  Bus Assignment : BusAssignment  AssignedSignals=HighBeamCmd,LowBeamCmd,LeftSignalCmd,RightSignalCmd,HazzardCmd
  Bus Creator1 : BusCreator  Inputs=6
  Compare To Constant : simulink/Logic and Bit Operations/Compare To Constant  relop===  const=3  OutDataTypeStr=boolean  ZeroCross=off
  Compare To Constant1 : simulink/Logic and Bit Operations/Compare To Constant  relop===  const=2  OutDataTypeStr=boolean  ZeroCross=off
  Compare To Constant2 : simulink/Logic and Bit Operations/Compare To Constant  relop===  const=-1  OutDataTypeStr=boolean  ZeroCross=off
  Compare To Constant3 : simulink/Logic and Bit Operations/Compare To Constant  relop===  const=1  OutDataTypeStr=boolean  ZeroCross=off
  Data Type Conversion : DataTypeConversion  SaturateOnIntegerOverflow=off  RndMeth=Floor
  Gear : Constant  Value=80  SampleTime=-1
  Hazzard : Constant  Value=0  OutDataTypeStr=boolean
  Headlights : Constant  Value=0
  IgnSwtch : Constant  Value=0
  Scaled Wheel Angle Limit [deg] : Gain  Gain=2*360/90
  Signal Lights : Constant  Value=0
  Signal Specification : SignalSpecification  Unit=1
  Signal Specification1 : SignalSpecification  Unit=1
  Signal Specification2 : SignalSpecification  Unit=1
  Signal Specification3 : SignalSpecification  Unit=deg
  Signal Specification4 : SignalSpecification  OutDataTypeStr=boolean  Unit=1
  Signal Specification5 : SignalSpecification  Unit=rad
  Steer : Constant  Value=0  SampleTime=-1
  To Virtual Bus : SignalConversion  ConversionOutput=Virtual bus  OverrideOpt=off
  Unit Conversion : UnitConversion
  VVCLightsCmd : Constant  Value=0  OutDataTypeStr=Bus: VVCLightsCmdBUS  SampleTime=-1
  Driver : Outport
  wires:
  Scaled Wheel Angle Limit [deg]/1 -> Signal Specification3/1
  Data Type Conversion/1 -> Signal Specification4/1
  Signal Specification4/1 -> Bus Creator1/5  "IgnSwtch"
  Bus Creator1/1 -> Driver/1
  Bus Assignment/1 -> To Virtual Bus/1
  Signal Specification5/1 -> Bus Creator1/1  "SteerCmd"
  Compare To Constant2/1 -> Bus Assignment/4
  Signal Specification3/1 -> Unit Conversion/1
  Gear/1 -> Signal Specification2/1
  To Virtual Bus/1 -> Bus Creator1/6  "LightsCmd"
  Brake/1 -> Signal Specification1/1
  Hazzard/1 -> Bus Assignment/6
  Signal Lights/1 -> Compare To Constant2/1, Compare To Constant3/1
  Signal Specification2/1 -> Bus Creator1/4  "GearCmd"
  Compare To Constant3/1 -> Bus Assignment/5
  VVCLightsCmd/1 -> Bus Assignment/1  "LightsCmd"
  Compare To Constant/1 -> Bus Assignment/2
  Unit Conversion/1 -> Signal Specification5/1
  Accelerator/1 -> Signal Specification/1
  IgnSwtch/1 -> Data Type Conversion/1
  Headlights/1 -> Compare To Constant/1, Compare To Constant1/1
  Steer/1 -> Scaled Wheel Angle Limit [deg]/1
  Signal Specification1/1 -> Bus Creator1/3  "DecelCmd"
  Signal Specification/1 -> Bus Creator1/2  "AccelCmd"
  Compare To Constant1/1 -> Bus Assignment/3

== system HEVminiproject/Driver Commands/Driver Commands/Game Wheel Hardware/Paddle Shift ==
  Buttons : Inport
  Add1 : Sum  Inputs=+-+
  Current Gear : UnitDelay  SampleTime=-1
  Data Type Conversion2 : DataTypeConversion  OutDataTypeStr=double  SaturateOnIntegerOverflow=off  RndMeth=Floor
  Demux2 : Demux  Outputs=2
  Detect Increase2 : simulink/Logic and Bit Operations/Detect Increase  vinit=0.0  OutDataTypeStr=boolean
  Logical Operator1 : Logic  Operator=XOR  Inputs=1  AllPortsSameDT=off  OutDataTypeStr=boolean
  Min/Max Gear : Saturate  UpperLimit=10  LowerLimit=-1
  Selector : Selector  InputPortWidth=32  IndexOptions=Index vector (dialog)  Indices=[5 6]  OutputSizes=1
  Switch2 : Switch  Criteria=u2 > Threshold  SaturateOnIntegerOverflow=off  InputSameDT=off
  Gear : Outport  VectorParamsAs1DForOutWhenUnconnected=off
  wires:
  Selector/1 -> Detect Increase2/1
  Buttons/1 -> Selector/1
  Min/Max Gear/1 -> Switch2/1
  Logical Operator1/1 -> Switch2/2
  Detect Increase2/1 -> Logical Operator1/1, Data Type Conversion2/1
  Data Type Conversion2/1 -> Demux2/1
  Demux2/2 -> Add1/2
  Demux2/1 -> Add1/1
  Switch2/1 -> Current Gear/1, Gear/1  "Gear"
  Current Gear/1 -> Switch2/3, Add1/3
  Add1/1 -> Min/Max Gear/1

== system HEVminiproject/Driver Commands/Driver Commands/Game Wheel Hardware/Stick Shift ==
  Buttons : Inport
  Gain : Gain  Gain=[-1 1:6]
  Selector1 : Selector  InputPortWidth=32  IndexOptions=Index vector (dialog)  Indices=[12:18]  OutputSizes=1
  Sum : Sum  Inputs=+
  Gear : Outport  VectorParamsAs1DForOutWhenUnconnected=off
  wires:
  Sum/1 -> Gear/1
  Buttons/1 -> Selector1/1
  Gain/1 -> Sum/1
  Selector1/1 -> Gain/1

== system HEVminiproject/Driver Commands/Driver Commands/Longitudinal Driver/Hill Hold & Stop ==
  LngRef : Inport
  <EnblDecelCmd> : Inport  Port=2
  <DecelOvrCmd> : Inport  Port=3
  <DecelHld> : Inport  Port=4
  <DecelZero> : Inport  Port=5
  Env : Inport  Port=6
  VehFdbk : Inport  Port=7
  Bus Selector : BusSelector  OutputSignals=Engine.EngSpdOut,Body.BdyFrm.Cg.Vel.xdot,Battery.BattInfo.BattSoc
  Bus Selector1 : BusSelector  OutputSignals=Body.BdyFrm.Cg.Vel.xdot
  Bus Selector2 : BusSelector  OutputSignals=Grade
  Hill Hold : Subsystem
  Logical Operator4 : Logic  Operator=OR  AllPortsSameDT=off  OutDataTypeStr=boolean
  Max : MinMax  Function=max  Inputs=2  ZeroCross=off
  Stop Detection : Subsystem
  Switch : Switch  Criteria=u2 > Threshold  SaturateOnIntegerOverflow=off  InputSameDT=off
  Switch1 : Switch  Criteria=u2 > Threshold  SaturateOnIntegerOverflow=off  InputSameDT=off
  VehFdbk1 : InportShadow  Port=7
  EnblDecelOvr : Outport
  DecelOvrCmd : Outport  Port=2
  DecelHld : Outport  Port=3
  DecelZero : Outport  Port=4
  VelFdbk : Outport  Port=5
  Grade : Outport  Port=6
  wires:
  Hill Hold/1(DecelOvr) -> Logical Operator4/1
  Hill Hold/2(EnblDecelOvr) -> Max/1
  Bus Selector/3 -> Hill Hold/3(<BattSoc>)  "<BattSoc>"
  Bus Selector/2 -> Hill Hold/2(<xdot>)  "<xdot>"
  Bus Selector/1 -> Hill Hold/1(<EngSpdOut>)  "<EngSpdOut>"
  Stop Detection/1(DecelOvrCmd) -> Max/2
  Stop Detection/2(EnblDecelOvr) -> Logical Operator4/2
  Logical Operator4/1 -> Switch/3
  Switch1/1 -> DecelOvrCmd/1
  Switch/1 -> EnblDecelOvr/1
  <EnblDecelCmd>/1 -> Switch1/2, Switch/1, Switch/2
  Max/1 -> Switch1/3
  Bus Selector1/1 -> VelFdbk/1, Stop Detection/2(<xdot>)  "<xdot>"
  LngRef/1 -> Hill Hold/4(LngRef), Stop Detection/1(LngRef)
  VehFdbk/1 -> Bus Selector/1
  <DecelOvrCmd>/1 -> Switch1/1
  Env/1 -> Bus Selector2/1
  Bus Selector2/1 -> Hill Hold/5(<Grade>), Grade/1  "<Grade>"
  VehFdbk1/1 -> Bus Selector1/1
  <DecelZero>/1 -> DecelZero/1
  <DecelHld>/1 -> DecelHld/1

== system HEVminiproject/Driver Commands/Driver Commands/Longitudinal Driver/Longitudinal Driver ==
  VelRef : Inport  Unit=m/s
  EnblAccelOvr : Inport  Port=2
  AccelOvrCmd : Inport  Port=3
  AccelHld : Inport  Port=4
  AccelZero : Inport  Port=5
  EnblDecelOvr : Inport  Port=6
  DecelOvrCmd : Inport  Port=7
  DecelHld : Inport  Port=8
  DecelZero : Inport  Port=9
  VelFdbk : Inport  Port=10  Unit=m/s
  Grade : Inport  Port=11
  ExtGearGround : Ground
  External Action Routing : Subsystem
  Longitudinal Driver : autolibsharedcommon/Longitudinal Driver  cntrlType=PI  shftType=Reverse, Neutral, Drive  vnom=vnom  Kp=Kp  Ki=Ki  Kaw=Kaw  Kff=Kff  Kg=Kg  tauerr=tauerr  tShift=tShift  tRev=tRev  tPark=tPark  pdlVec=pdlVec  upShftTbl=upShftTbl  dwnShftTbl=dwnShftTbl  GearInit=GearInit  tClutch=tClutch  VehVelVec=VehVelVec  KffVec=KffVec  KiVec=KiVec  KpVec=KpVec  KgVec=KgVec  m=m  Kpt=Kpt  Lvv=L  g=g  UpGearVec=UpGearVec  DownGearVec=DownGearVec  aMode=6  errUnit=m/s  aR=aR  bR=bR  cR=cR  tauPt=tauPt
      settings: LibrarySourceBlock=autolibshared/Longitudinal Driver/Longitudinal Driver
  Info : Outport  InitialOutput=0  VectorParamsAs1DForOutWhenUnconnected=off
  AccelCmd : Outport  Port=2  VectorParamsAs1DForOutWhenUnconnected=off
  DecelCmd : Outport  Port=3  VectorParamsAs1DForOutWhenUnconnected=off
  GearCmd : Outport  Port=4
  wires:
  DecelZero/1 -> External Action Routing/8(DecelZero)
  DecelHld/1 -> External Action Routing/7(DecelHld)
  DecelOvrCmd/1 -> External Action Routing/6(DecelOvrCmd)
  EnblDecelOvr/1 -> External Action Routing/5(EnblDecelOvr)
  AccelZero/1 -> External Action Routing/4(AccelZero)
  AccelHld/1 -> External Action Routing/3(AccelHld)
  AccelOvrCmd/1 -> External Action Routing/2(AccelOvrCmd)
  EnblAccelOvr/1 -> External Action Routing/1(EnblAccelOvr)
  Longitudinal Driver/4 -> GearCmd/1
  ExtGearGround/1 -> Longitudinal Driver/4
  External Action Routing/1(ExtActions) -> Longitudinal Driver/5
  Grade/1 -> Longitudinal Driver/3
  Longitudinal Driver/3 -> DecelCmd/1
  Longitudinal Driver/2 -> AccelCmd/1
  Longitudinal Driver/1 -> Info/1
  VelFdbk/1 -> Longitudinal Driver/2
  VelRef/1 -> Longitudinal Driver/1

== system HEVminiproject/Driver Commands/Driver Commands/Predictive Driver/Hill Hold & Stop ==
  LngRef : Inport
  <EnblDecelCmd> : Inport  Port=2
  <DecelOvrCmd> : Inport  Port=3
  <DecelHld> : Inport  Port=4
  <DecelZero> : Inport  Port=5
  Env : Inport  Port=6
  VehFdbk : Inport  Port=7
  Bus Selector : BusSelector  OutputSignals=Engine.EngSpdOut,Body.BdyFrm.Cg.Vel.xdot,Battery.BattInfo.BattSoc
  Bus Selector1 : BusSelector  OutputSignals=Body.BdyFrm.Cg.Vel.xdot
  Bus Selector2 : BusSelector  OutputSignals=Grade
  Hill Hold : Subsystem
  Logical Operator4 : Logic  Operator=OR  AllPortsSameDT=off  OutDataTypeStr=boolean
  Max : MinMax  Function=max  Inputs=2
  Stop Detection : Subsystem
  Switch : Switch  Criteria=u2 > Threshold  SaturateOnIntegerOverflow=off  InputSameDT=off
  Switch1 : Switch  Criteria=u2 > Threshold  SaturateOnIntegerOverflow=off  InputSameDT=off
  VehFdbk1 : InportShadow  Port=7
  EnblDecelOvr : Outport
  DecelOvrCmd : Outport  Port=2
  DecelHld : Outport  Port=3
  DecelZero : Outport  Port=4
  Grade : Outport  Port=5
  VelFdbk : Outport  Port=6
  wires:
  Hill Hold/1(DecelOvr) -> Logical Operator4/1
  Hill Hold/2(EnblDecelOvr) -> Max/1
  Bus Selector/3 -> Hill Hold/3(<BattSoc>)  "<BattSoc>"
  Bus Selector/2 -> Hill Hold/2(<xdot>)  "<xdot>"
  Bus Selector/1 -> Hill Hold/1(<EngSpdOut>)  "<EngSpdOut>"
  Stop Detection/1(DecelOvrCmd) -> Max/2
  Stop Detection/2(EnblDecelOvr) -> Logical Operator4/2
  Logical Operator4/1 -> Switch/3
  Switch1/1 -> DecelOvrCmd/1
  Switch/1 -> EnblDecelOvr/1
  <EnblDecelCmd>/1 -> Switch1/2, Switch/1, Switch/2
  Max/1 -> Switch1/3
  Bus Selector1/1 -> VelFdbk/1, Stop Detection/2(<xdot>)  "<xdot>"
  LngRef/1 -> Hill Hold/4(LngRef), Stop Detection/1(LngRef)
  VehFdbk/1 -> Bus Selector/1
  <DecelOvrCmd>/1 -> Switch1/1
  Env/1 -> Bus Selector2/1
  Bus Selector2/1 -> Hill Hold/5(<Grade>), Grade/1  "<Grade>"
  VehFdbk1/1 -> Bus Selector1/1
  <DecelZero>/1 -> DecelZero/1
  <DecelHld>/1 -> DecelHld/1

== system HEVminiproject/Driver Commands/Driver Commands/Predictive Stanley Driver/Hill Hold & Stop ==
  LngRef : Inport
  <EnblDecelCmd> : Inport  Port=2
  <DecelOvrCmd> : Inport  Port=3
  <DecelHld> : Inport  Port=4
  <DecelZero> : Inport  Port=5
  <CurvRef> : Inport  Port=6
  Env : Inport  Port=7
  VehFdbk : Inport  Port=8
  Bus Selector : BusSelector  OutputSignals=Engine.EngSpdOut,Body.BdyFrm.Cg.Vel.xdot,Battery.BattInfo.BattSoc
  Bus Selector1 : BusSelector  OutputSignals=Body.BdyFrm.Cg.Vel.xdot
  Bus Selector2 : BusSelector  OutputSignals=Grade
  Hill Hold : Subsystem
  Logical Operator4 : Logic  Operator=OR  AllPortsSameDT=off  OutDataTypeStr=boolean
  Max : MinMax  Function=max  Inputs=2
  Stop Detection : Subsystem
  Switch : Switch  Criteria=u2 > Threshold  SaturateOnIntegerOverflow=off  InputSameDT=off
  Switch1 : Switch  Criteria=u2 > Threshold  SaturateOnIntegerOverflow=off  InputSameDT=off
  VehFdbk1 : InportShadow  Port=8
  EnblDecelOvr : Outport
  DecelOvrCmd : Outport  Port=2
  DecelHld : Outport  Port=3
  DecelZero : Outport  Port=4
  Grade : Outport  Port=5
  CurvRef : Outport  Port=6
  VelFdbk : Outport  Port=7
  wires:
  Hill Hold/1(DecelOvr) -> Logical Operator4/1
  Hill Hold/2(EnblDecelOvr) -> Max/1
  Bus Selector/3 -> Hill Hold/3(<BattSoc>)  "<BattSoc>"
  Bus Selector/2 -> Hill Hold/2(<xdot>)  "<xdot>"
  Bus Selector/1 -> Hill Hold/1(<EngSpdOut>)  "<EngSpdOut>"
  Stop Detection/1(DecelOvrCmd) -> Max/2
  Stop Detection/2(EnblDecelOvr) -> Logical Operator4/2
  Logical Operator4/1 -> Switch/3
  Switch1/1 -> DecelOvrCmd/1
  Switch/1 -> EnblDecelOvr/1
  <EnblDecelCmd>/1 -> Switch1/2, Switch/1, Switch/2
  Max/1 -> Switch1/3
  Bus Selector1/1 -> VelFdbk/1, Stop Detection/2(<xdot>)  "<xdot>"
  LngRef/1 -> Hill Hold/4(LngRef), Stop Detection/1(LngRef)
  <CurvRef>/1 -> CurvRef/1
  VehFdbk/1 -> Bus Selector/1
  <DecelOvrCmd>/1 -> Switch1/1
  Env/1 -> Bus Selector2/1
  Bus Selector2/1 -> Hill Hold/5(<Grade>), Grade/1  "<Grade>"
  VehFdbk1/1 -> Bus Selector1/1
  <DecelZero>/1 -> DecelZero/1
  <DecelHld>/1 -> DecelHld/1

== system HEVminiproject/Environment/Ground Feedback/3D Terrain/3D Engine Source ==
  WheelFdbk : Inport
  Multiple Points : Subsystem  VariantControl=terrType==2
  Single Point : Subsystem  VariantControl=terrType ==1
  z : Outport
  DCM : Outport  Port=2

== system HEVminiproject/Environment/Ground Feedback/Height Map/2D Lookup Tbl for Elevation, Z ==
  XWhl : Inport  Partition=on  PartitionDimension=1  PartitionWidth=1  PartitionOffset=0
  YWhl : Inport  Port=2  Partition=on  PartitionDimension=1  PartitionWidth=1  PartitionOffset=0
  2-D Lookup Table : Lookup_n-D  BreakpointsForDimension1=EnvScnHeightMapXBpts  BreakpointsForDimension2=EnvScnHeightMapYBpts  BeginIndexSearchUsingPreviousIndexResult=on  Table=EnvScnHeightMap  ExtrapMethod=Clip  InternalRulePriority=Speed  RndMeth=Simplest
      settings: InputPortMap=u0,u1
  Add : Sum
  Add1 : Sum
  Constant : Constant  Value=0
  Constant1 : Constant  Value=0
  For Each : ForEach  DisableCoverage=on
  Unary Minus : UnaryMinus
  Z : Outport  ConcatenationDimension=1
  wires:
  2-D Lookup Table/1 -> Z/1
  YWhl/1 -> Unary Minus/1
  XWhl/1 -> Add1/2
  Unary Minus/1 -> Add/1
  Add/1 -> 2-D Lookup Table/2
  Constant/1 -> Add/2
  Constant1/1 -> Add1/1
  Add1/1 -> 2-D Lookup Table/1

== system HEVminiproject/Environment/Ground Feedback/Height Map/Wheel Coordinates ==
  FrntAxlLftX : Inport
  FrntAxlRghtX : Inport  Port=2
  RearAxlLftX : Inport  Port=3
  RearAxlRghtX : Inport  Port=4
  FrntAxlLftY : Inport  Port=5
  FrntAxlRghtY : Inport  Port=6
  RearAxlLftY : Inport  Port=7
  RearAxlRghtY : Inport  Port=8
  Matrix Concatenate : Concatenate  NumInputs=4  Mode=Multidimensional array
  Matrix Concatenate1 : Concatenate  NumInputs=4  Mode=Multidimensional array
  XWhl : Outport
  YWhl : Outport  Port=2
  wires:
  Matrix Concatenate1/1 -> YWhl/1
  FrntAxlLftX/1 -> Matrix Concatenate/1
  FrntAxlLftY/1 -> Matrix Concatenate1/1
  FrntAxlRghtY/1 -> Matrix Concatenate1/2
  FrntAxlRghtX/1 -> Matrix Concatenate/2
  RearAxlLftY/1 -> Matrix Concatenate1/3
  RearAxlLftX/1 -> Matrix Concatenate/3
  RearAxlRghtY/1 -> Matrix Concatenate1/4
  Matrix Concatenate/1 -> XWhl/1
  RearAxlRghtX/1 -> Matrix Concatenate/4

== system HEVminiproject/Environment/Ground Feedback/Inclined Plane/Ideal Inclined Plane ==
  X : Inport
  Y : Inport  Port=2
  phi : Inport  Port=3
  theta : Inport  Port=4
  Constant : Constant  Value=Z_est
  Enabled : Subsystem  Variant=on
  Signal Specification1 : SignalSpecification  Unit=rad
  Signal Specification3 : SignalSpecification  Unit=rad
  Signal Specification4 : SignalSpecification  Unit=m
  Signal Specification5 : SignalSpecification  Unit=m
  Signal Specification6 : SignalSpecification  Unit=m
  Z Plane : MATLAB Function  InitFcn=|  TreatAsAtomicUnit=on
      | if builtin('license','test','Vehicle_Dynamics_Blockset')
      |    [~]=builtin('license','checkout','Vehicle_Dynamics_Blockset');
      | else
      |    error(message('autoblks_shared:autosharederrAutoIcon:invalidLicense'));
      | end
      mask init:
      | if builtin('license','test','Vehicle_Dynamics_Blockset')
      |     [~]=builtin('license','checkout','Vehicle_Dynamics_Blockset');
      | else
      |     error(message('autoblks_shared:autosharederrAutoIcon:invalidLicense'));
      | end
  Z : Outport
  DCM : Outport  Port=2
  wires:
  Z Plane/2(DCM) -> DCM/1
  Signal Specification1/1 -> Z Plane/5(theta), Enabled/3(theta)
  phi/1 -> Signal Specification3/1
  theta/1 -> Signal Specification1/1
  Signal Specification3/1 -> Z Plane/4(phi), Enabled/2(phi)
  Y/1 -> Signal Specification6/1
  Z Plane/1(Z) -> Signal Specification4/1
  X/1 -> Signal Specification5/1
  Signal Specification4/1 -> Z/1
  Signal Specification5/1 -> Z Plane/1(X)
  Signal Specification6/1 -> Z Plane/2(Y)
  Constant/1 -> Enabled/1(Z), Z Plane/3(Zoffset)

== system HEVminiproject/Environment/Ground Feedback/Inclined Plane/Wheel Coordinates ==
  FrntAxlLftX : Inport
  FrntAxlRghtX : Inport  Port=2
  RearAxlLftX : Inport  Port=3
  RearAxlRghtX : Inport  Port=4
  FrntAxlLftY : Inport  Port=5
  FrntAxlRghtY : Inport  Port=6
  RearAxlLftY : Inport  Port=7
  RearAxlRghtY : Inport  Port=8
  Matrix Concatenate : Concatenate  NumInputs=4  Mode=Multidimensional array
  Matrix Concatenate1 : Concatenate  NumInputs=4  Mode=Multidimensional array
  XWhl : Outport
  YWhl : Outport  Port=2
  wires:
  RearAxlRghtX/1 -> Matrix Concatenate/4
  Matrix Concatenate/1 -> XWhl/1
  RearAxlRghtY/1 -> Matrix Concatenate1/4
  RearAxlLftX/1 -> Matrix Concatenate/3
  RearAxlLftY/1 -> Matrix Concatenate1/3
  FrntAxlRghtX/1 -> Matrix Concatenate/2
  FrntAxlRghtY/1 -> Matrix Concatenate1/2
  FrntAxlLftY/1 -> Matrix Concatenate1/1
  FrntAxlLftX/1 -> Matrix Concatenate/1
  Matrix Concatenate1/1 -> YWhl/1
